simulink model "ConvertUnitRpm"  (R2021b)
settings: Solver=FixedStepAuto  StartTime=0.0  StopTime=10.0  FixedStep=0.2  RelTol=1e-3
libraries: simulink x1
settings Model: Creator=ajfem  LastModifiedBy=ajfem

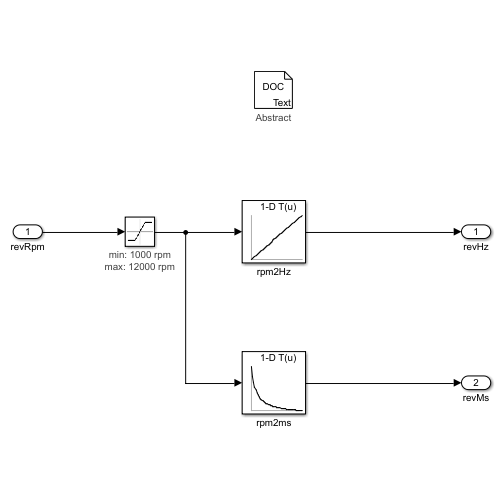
[thumbnail: Simulink's stored preview of the top-level diagram]
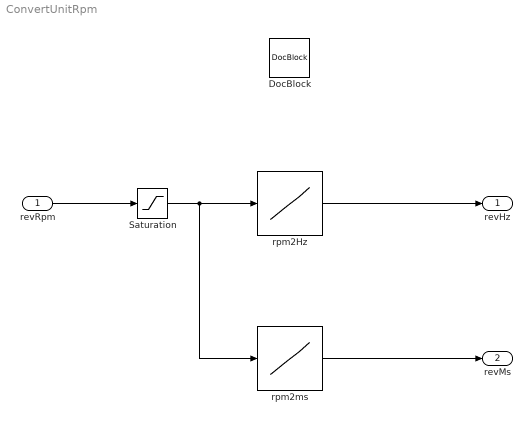
== system ConvertUnitRpm ==
  revRpm : Inport  OutDataTypeStr=double  Unit=rpm  PortDimensions=1
  DocBlock : simulink/Model-Wide Utilities/DocBlock  ECoderFlag=Abstract  DocumentType=Text
      content=|
      | This model converts rpm decimal values to Hz and ms.
      | Hz conversion is linear and it´s quite robust.
      | ms conversion is not so good at low rpms away from breakpoints.
      settings: AttributesFormatString=%<ECoderFlag>
  Saturation : Saturate  UpperLimit=12000  LowerLimit=1000
      settings: AttributesFormatString=|
      | min: %<LowerLimit> rpm
      | max: %<UpperLimit> rpm
  rpm2Hz : Lookup_n-D  NumberOfTableDimensions=1  BreakpointsForDimension1=[1000:250:12000]  Table=[1000:250:12000]/60  InternalRulePriority=Speed  RndMeth=Simplest  InputSameDT=on
  rpm2ms : Lookup_n-D  NumberOfTableDimensions=1  BreakpointsForDimension1=[1000:250:12000]  Table=60*1000./[1000:250:12000]  InternalRulePriority=Speed  RndMeth=Simplest  InputSameDT=on
  revHz : Outport  OutDataTypeStr=double  Unit=Hz  PortDimensions=1
  revMs : Outport  Port=2  OutDataTypeStr=double  Unit=msec  PortDimensions=1
  wires:
  revRpm/1 -> Saturation/1
  rpm2Hz/1 -> revHz/1
  Saturation/1 -> rpm2ms/1, rpm2Hz/1
  rpm2ms/1 -> revMs/1
